simulink model "rayTrace_th"  (R2018b)
settings: Solver=FixedStepAuto  StartTime=0.0  StopTime=0  FixedStep=1  RelTol=1e-3
undefined symbols (not defined in the file or in its folder): pitch_deg, pixelCol, pixelRow, roll_deg, yaw_deg
libraries: rayTrace_ul x1
settings Model: Creator=mcobb  LastModifiedBy=mcobb

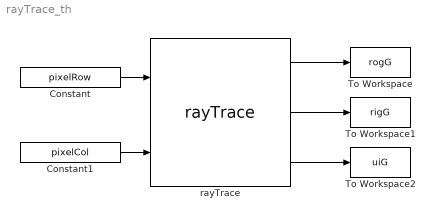
== system rayTrace_th ==
  Constant : Constant  Value=pixelRow
  Constant1 : Constant  Value=pixelCol
  To Workspace : ToWorkspace  VariableName=rogG  SaveFormat=Timeseries  SampleTime=-1
  To Workspace1 : ToWorkspace  VariableName=rigG  SaveFormat=Timeseries  SampleTime=-1
  To Workspace2 : ToWorkspace  VariableName=uiG  SaveFormat=Timeseries  SampleTime=-1
  rayTrace : rayTrace_ul/rayTrace  camPosVec_cm=camPosVec_cm  camEulAngles_deg=[roll_deg pitch_deg yaw_deg]  dist2Glass_cm=dist2Glass_cm  indOfRefVec=indOfRefVec  glassPlane=glassPlane  glassThickness_cm=glassThickness_cm  imageDimsVec_px=imageDims_px  camFOV_deg=cameraFOV_deg
  wires:
  Constant/1 -> rayTrace/1
  Constant1/1 -> rayTrace/2
  rayTrace/1 -> To Workspace/1
  rayTrace/3 -> To Workspace2/1
  rayTrace/2 -> To Workspace1/1
